simulink model "microturbine_model_v2"  (R2025b)
settings: Solver=ode4  StartTime=0.0  StopTime=inf  FixedStep=0.002  RelTol=1e-3
values from neighbouring files (symbols this model uses):
  c_p_air = 1005    [data_v2.m]
  c_p_eg = 1100    [data_v2.m]
  c_p_w = 4184    [data_v2.m]
  dp = dp_run    [data_v2.m]
  eps_HRB = 0.75    [data_v2.m]
  eta_c = 0.81    [data_v2.m]
  eta_comb = 0.99    [data_v2.m]
  eta_gen = 0.98    [data_v2.m]
  eta_mech = 0.97    [data_v2.m]
  eta_t = 0.88    [data_v2.m]
  hot_water_setpoint = 60    [data_v2.m]
  J = 3e-3    (= 0.003)    [data_v2.m]
  k_air = 1.4    [data_v2.m]
  lambda = 0.313    [data_v2.m]
  lambda_eg_filter = 15e3    (= 15000)    [data_v2.m]
  LHV = 47e6    (= 47000000)    [data_v2.m]
  M_buffer = 20    [data_v2.m]
  P0 = dp.power.P_el    [data_v2.m]
  P1 = P_amb - filter_P    (= 100325)    [data_v2.m]
  P_amb = 101325    [data_v2.m]
  P_el_max = 0.95 * max(sched.P_el_W)    [data_v2.m]
  P_el_min = 1.1 * polyval(fitPmin, T1 - 273.15) * 1e3    [data_v2.m]
  R_air = c_p_air * (k_air-1)/k_air    (= 287.142857143)    [data_v2.m]
  sched = sched_run    [data_v2.m]
  T1 = T1_run    (= 288.15)    [data_v2.m]
  T3_max = 960+273.15    (= 1233.15)    [data_v2.m]
  T3_min = 650+273.15    (= 923.15)    [data_v2.m]
  T_cold_water = 15    [data_v2.m]
  V = 0.025    [data_v2.m]
libraries: nesl_utility x4, simulink x3, slpidlib x2, fl_lib x1
settings Model: Creator=Alessandro  LastModifiedBy=Alessandro

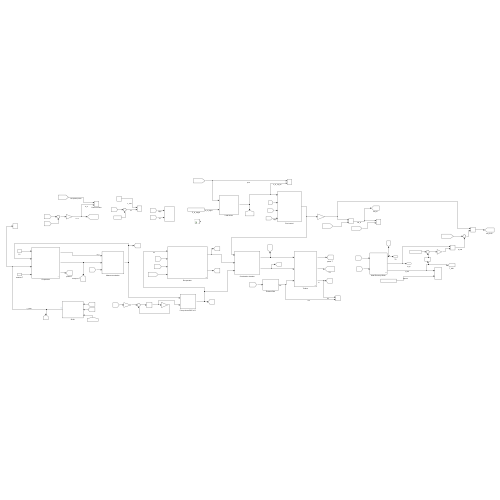
[thumbnail: Simulink's stored preview of the top-level diagram]
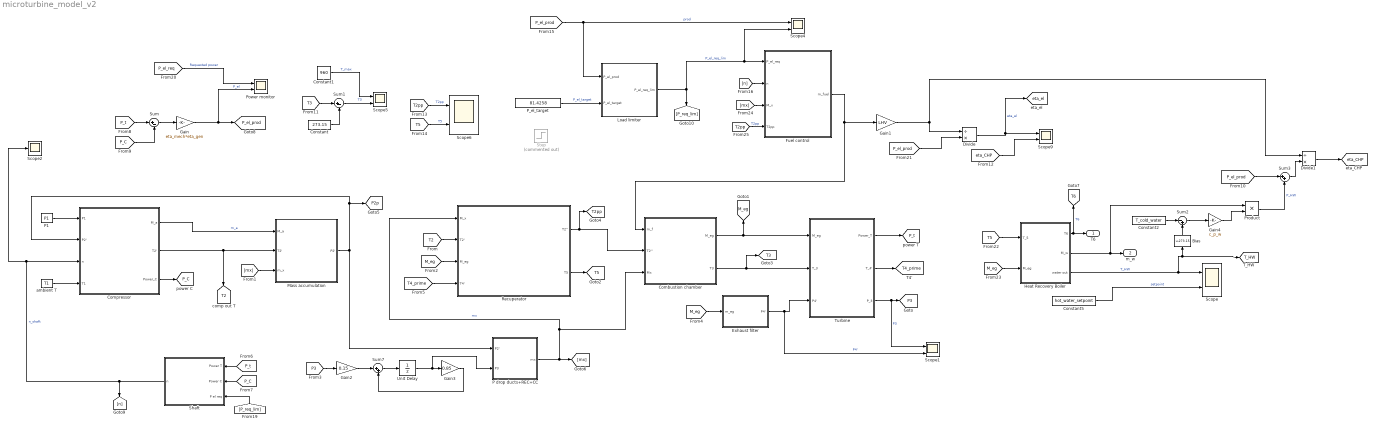
== system microturbine_model_v2 ==
  Bias : Bias  Bias=-273.15  SaturateOnIntegerOverflow=off
  Combustion chamber : Subsystem
      mask Display: image('360_F_235263034_miJw2igmixo7ymCqhHZ7c8wp9kaujzfM.jpg');
  Compressor : Subsystem
      mask Display: image('compressor_icon.png');
  Constant : Constant  Value=273.15
  Constant1 : Constant  Value=960
  Constant2 : Constant  Value=T_cold_water
  Constant5 : Constant  Value=hot_water_setpoint
  Divide : Product  Inputs=/*
  Divide1 : Product  Inputs=/*
  Exhaust filter : Subsystem
  Fuel control : Subsystem
  Gain : Gain  Gain=eta_mech*eta_gen
  Gain1 : Gain  Gain=LHV
  Gain2 : Gain  Gain=0.15
  Gain3 : Gain  Gain=0.85
  Gain4 : Gain  Gain=c_p_w
  Heat Recovery Boiler : Subsystem
  Load limiter : Subsystem
  Mass accumulation : Subsystem
  P drop ducts+REC+CC : Subsystem
  P1 : Constant  Value=P1
  P_el_target : Constant  Value=81.4258
  Power monitor : Scope  NumInputPorts=2
      settings: ActiveDisplayYMinimum=-9170.58872046804  ActiveDisplayYMaximum=119683.00366407538  DataLoggingDecimation=50  DataLoggingVariableName=ScopeData7
  Product : Product
  Recuperator : Subsystem
      mask Display: image('Heat-Transfer-in-a-Double-Pipe-Heat-Exchanger.jpg');
  Scope{,1,4..6,9} (6 alike) : Scope  NumInputPorts=2
      Scope settings: ActiveDisplayYMinimum=3.191503786041018  ActiveDisplayYMaximum=105.72122088980728  DataLoggingDecimation=50
      Scope1 settings: TimeDisplayOffset=20  ActiveDisplayYMinimum=-67410.697407891537  ActiveDisplayYMaximum=604536.71720488416  DataLoggingDecimation=50
      Scope4 settings: ActiveDisplayYMinimum=72643.782114693779  ActiveDisplayYMaximum=83704.868974122015  DataLoggingDecimation=50  DataLoggingVariableName=ScopeData8
      Scope5 settings: ActiveDisplayYMinimum=954.15751527655459  ActiveDisplayYMaximum=959.34960531631691  DataLoggingDecimation=50  DataLoggingVariableName=ScopeData5
      Scope6 settings: ActiveDisplayYMinimum=549.25379795566278  ActiveDisplayYMaximum=874.2834530892867  DataLoggingDecimation=50  DataLoggingVariableName=ScopeData6
      Scope9 settings: ActiveDisplayYMinimum=0.15948540822321575  ActiveDisplayYMaximum=0.4992395185212698  DataLoggingDecimation=50  DataLoggingVariableName=ScopeData9
  Scope2 : Scope
      settings: ActiveDisplayYMinimum=40436.974761073478  ActiveDisplayYMaximum=81944.16250433313  DataLoggingDecimation=50  DataLoggingVariableName=ScopeData2
  Shaft : Subsystem
  Step : Step  Commented=on  Time=10  Before=P0  After=P_el_max  SampleTime=0
  Sum : Sum  Inputs=|+-
  Sum1 : Sum  Inputs=|+-
  Sum2 : Sum  Inputs=|-+
  Sum3 : Sum  Inputs=|++
  Sum7 : Sum  Inputs=|++
  Turbine : Subsystem
  Unit Delay : UnitDelay  InitialCondition=dp.stations(3).P  SampleTime=-1  HasFrameUpgradeWarning=on
  ambient T : Constant  Value=T1
  T6 : Outport
  m_w : Outport  Port=2
  tag scope: M_eg=global, P2p=global, P3=global, P_C=global, P_el_prod=global, P_t=global, T2=global, T2pp=global, T3=global, T4_prime=global, T5=global, T6=global, T_HW=global, eta_CHP=global, eta_el=global
  wires:
  Compressor/1(M_a) -> Mass accumulation/1(M_a)  "m_a"
  Mass accumulation/1(P2') -> Compressor/2(P2'), [P2p], P drop ducts+REC+CC/1(P2')
  Compressor/2(T2') -> Mass accumulation/2(T2'), [T2]
  P1/1 -> Compressor/1(P1)
  [T2] -> Recuperator/2(T2')
  Recuperator/1(T2'') -> [T2pp], Combustion chamber/2("T2'' ")
  Combustion chamber/1("M_eg ") -> [M_eg], Turbine/1(M_eg)
  [M_eg] -> Recuperator/3(M_eg)
  Recuperator/2(T5) -> [T5]
  Combustion chamber/2(T3) -> [T3], Turbine/2(T_3)
  Turbine/3(P_3) -> Scope1/1, [P3]  "P3"
  Exhaust filter/1(P4') -> Scope1/2, Turbine/3(P4')  "P4'"
  [M_eg] -> Exhaust filter/1(m_eg)
  Compressor/3(Power_C) -> [P_C]
  [P_t] -> Shaft/1(Power T)
  [P_C] -> Shaft/2(Power C)
  [P_t] -> Sum/1
  [P_C] -> Sum/2
  Sum/1 -> Gain/1
  Gain/1 -> [P_el_prod], Power monitor/2  "P_el"
  P drop ducts+REC+CC/1(mx) -> [mx], Combustion chamber/3(Mx), Recuperator/1(M_x)  "mx"
  [mx] -> Mass accumulation/3(m_x)
  Fuel control/1(m_fuel) -> Combustion chamber/1(m_f), Gain1/1
  [P3] -> Gain2/1
  [T4_prime] -> Recuperator/4(T4')
  Turbine/2(T_4') -> [T4_prime]
  Turbine/1(Power_T) -> [P_t]
  Gain2/1 -> Sum7/1
  Unit Delay/1 -> P drop ducts+REC+CC/2(P3), Gain3/1
  Gain3/1 -> Sum7/2
  Sum7/1 -> Unit Delay/1
  [P_req_lim] -> Shaft/3(P el req)
  [T2pp] -> Scope6/1  "T2pp"
  [T5] -> Scope6/2  "T5"
  [T3] -> Sum1/1
  Sum1/1 -> Scope5/2  "T3"
  Constant/1 -> Sum1/2
  Constant1/1 -> Scope5/1  "T_max"
  [P_el_prod] -> Divide/2
  Gain1/1 -> Divide/1, Divide1/1
  Divide/1 -> [eta_el], Scope9/1  "eta_el"
  ambient T/1 -> Compressor/4(T1)
  [T5] -> Heat Recovery Boiler/1(T_5)
  [M_eg] -> Heat Recovery Boiler/2(M_eg)
  Heat Recovery Boiler/1(T6) -> T6/1, [T6]  "T6"
  Heat Recovery Boiler/2(M_w) -> Product/1, m_w/1
  Heat Recovery Boiler/3(water out) -> Bias/1, [T_HW], Scope/1  "T_HW"
  Constant5/1 -> Scope/2  "setpoint"
  [P_el_req] -> Power monitor/1  "Requested power"
  [mx] -> Fuel control/3(M_x)
  [T2pp] -> Fuel control/4(T2pp)  "T2pp"
  [n] -> Fuel control/2(n)
  [P_el_prod] -> Load limiter/1(P_el_prod), Scope4/1  "prod"
  Shaft/1(n) -> Scope2/1, Compressor/3(n), [n]  "n_shaft"
  Load limiter/1(P_el_req_lim) -> [P_req_lim], Scope4/2, Fuel control/1(P_el_req)  "P_el_req_lim"
  P_el_target/1 -> Load limiter/2(P_el_target)  "P_el_target"
  Constant2/1 -> Sum2/1
  Sum2/1 -> Gain4/1
  Gain4/1 -> Product/2
  Product/1 -> Sum3/2  "P_HW"
  [P_el_prod] -> Sum3/1
  Sum3/1 -> Divide1/2
  Divide1/1 -> [eta_CHP]
  [eta_CHP] -> Scope9/2
  Bias/1 -> Sum2/2

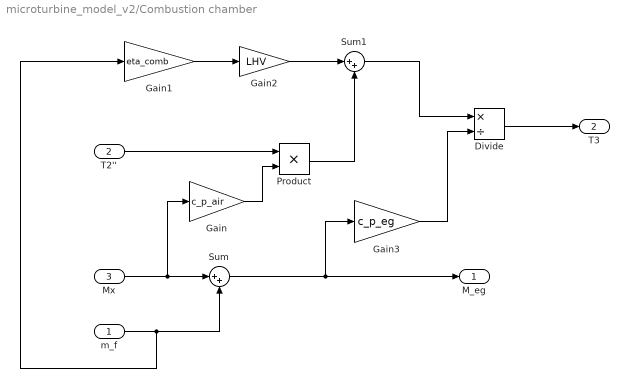
== system microturbine_model_v2/Combustion chamber ==
  m_f : Inport
  "T2'' " : Inport  Port=2
  Mx : Inport  Port=3
  Divide : Product  Inputs=*/
  Gain : Gain  Gain=c_p_air
  Gain1 : Gain  Gain=eta_comb
  Gain2 : Gain  Gain=LHV
  Gain3 : Gain  Gain=c_p_eg
  Product : Product
  Sum : Sum  Inputs=|++
  Sum1 : Sum  Inputs=|++
  "M_eg " : Outport
  T3 : Outport  Port=2
  wires:
  Sum/1 -> "M_eg "/1, Gain3/1
  Mx/1 -> Gain/1, Sum/1
  m_f/1 -> Sum/2, Gain1/1
  Sum1/1 -> Divide/1
  Divide/1 -> T3/1
  Gain/1 -> Product/2
  Gain1/1 -> Gain2/1
  Gain2/1 -> Sum1/1
  "T2'' "/1 -> Product/1
  Product/1 -> Sum1/2
  Gain3/1 -> Divide/2

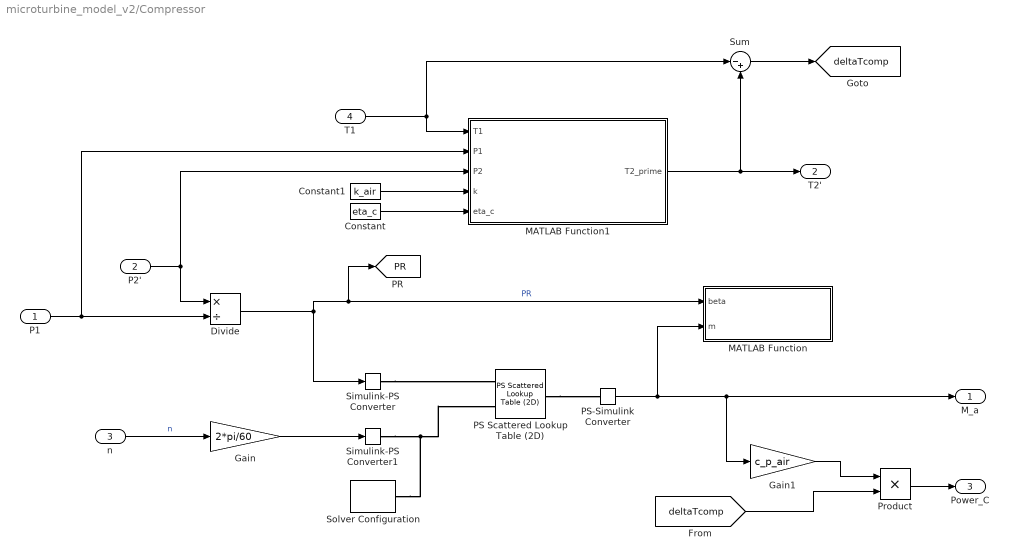
== system microturbine_model_v2/Compressor ==
  P1 : Inport
  P2' : Inport  Port=2
  n : Inport  Port=3
  T1 : Inport  Port=4
  Constant : Constant  Value=eta_c
  Constant1 : Constant  Value=k_air
  Divide : Product  Inputs=*/
  Gain : Gain  Gain=2*pi/60
  Gain1 : Gain  Gain=c_p_air
  MATLAB Function : MATLAB Function  TreatAsAtomicUnit=on
  MATLAB Function1 : MATLAB Function  TreatAsAtomicUnit=on
  PS Scattered Lookup Table (2D) : fl_lib/Physical Signals/Lookup Tables/PS Scattered Lookup Table (2D)  x1=beta  x2=n rad/s  f=flow kg/s  extrap_method=simscape.enum.extrapolation_slu.linear
      settings: InternalSimscapePortConfiguration="{\"Bottom\":[],\"Left\":[{\"id\":\"I1\",\"label\":\"x1\",\"type\":\"input\"},{\"id\":\"I2\",\"label\":\"x2\",\"type\":\"input\"}],\"Right\":[{\"id\":\"O\",\"label\":\"f\",\"type\":\"output\"}],\"Top\":[]}"
  PS-Simulink Converter : nesl_utility/PS-Simulink Converter  PhysicalDomain=network_engine_domain  SubClassName=ps_output  LeftPortType=input  RightPortType=output  PseudoPeriodic=off  Frequencies=[]  VectorFormat=inherit  Unit=inherit  AffineConversion=off
  Product : Product
  Simulink-PS Converter : nesl_utility/Simulink-PS Converter  PhysicalDomain=network_engine_domain  SubClassName=ps_input  LeftPortType=input  RightPortType=output  PseudoPeriodic=off  Frequencies=[]  NoiseDistribution=none  NoiseParameters=[]  Unit=1  AffineConversion=off  FilteringAndDerivatives=provide  SimscapeFilterOrder=1  InputFilterTimeConstant=0.001  UdotUserProvided=0
  Simulink-PS Converter1 : nesl_utility/Simulink-PS Converter  PhysicalDomain=network_engine_domain  SubClassName=ps_input  LeftPortType=input  RightPortType=output  PseudoPeriodic=off  Frequencies=[]  NoiseDistribution=none  NoiseParameters=[]  Unit=rad/s  AffineConversion=off  FilteringAndDerivatives=provide  SimscapeFilterOrder=1  InputFilterTimeConstant=0.001  UdotUserProvided=0
  Solver Configuration : nesl_utility/Solver Configuration  PhysicalDomain=network_engine_domain  SubClassName=solver  LeftPortType=input  RightPortType=generic  Tones=[]  Harmonics=[]  SimulateNoise=off  Profile=off  UseLocalSampling=off  EnableSwitchedLinearOptims=on  FrequencyDomain=off  UseCCode=off  RelTol=0.001  AbsTol=0.001  MinStep=1e-09  ToWorkspace=off  RevertToSquareIcSolve=off  NumHomotopyIterations=100  PhasorMode=off  PhasorModeNumHarmonics=1  ConsistencySolver=NEWTON_XTOL_AFTER_FTOL  IndexReductionMethod=DerivativeReplacement  DoDC=off  ResidualTolerance=1e-09  ConsistencyTolSource=GLOBAL  ConsistencyAbsTol=0.001  ConsistencyRelTol=0.001  ConsistencyTolFactor=0.001  UseLocalSolver=off  LocalSolverChoice=NE_BACKWARD_EULER_ADVANCER  ResolveIndetEquations=on  FunctionEvalNumThread=1  LocalSolverSampleTime=0.0001  DoFixedCost=off  MaxNonlinIter=3  MaxModeIter=2  ComputeImpulses=off  ImpulseIterations=2  LinearAlgebra=auto  LinearAlgebraNumThread=0  EquationFormulation=NE_TIME_EF  DelaysMemoryBudget=1024  AutomaticFiltering=on  FilteringTimeConstant=0.001  PartitionStorageMethod=AS_NEEDED  PartitionMemoryBudget=1024  PartitionMethod=ROBUST  MultibodyUseLocalSolver=off  MultibodyLocalSolverChoice=ODE1  MultibodyLocalSolverSampleTime=0.001
  Sum : Sum  Inputs=|-+
  M_a : Outport
  T2' : Outport  Port=2
  Power_C : Outport  Port=3
  tag scope: PR=global, deltaTcomp=global
  wires:
  PS-Simulink Converter/1 -> MATLAB Function/2(m), Gain1/1, M_a/1
  Gain/1 -> Simulink-PS Converter1/1
  n/1 -> Gain/1  "n"
  P2'/1 -> MATLAB Function1/3(P2), Divide/1
  P1/1 -> MATLAB Function1/2(P1), Divide/2
  Divide/1 -> Simulink-PS Converter/1, [PR], MATLAB Function/1(beta)  "PR"
  Constant1/1 -> MATLAB Function1/4(k)
  T1/1 -> MATLAB Function1/1(T1), Sum/1
  Constant/1 -> MATLAB Function1/5(eta_c)
  MATLAB Function1/1(T2_prime) -> Sum/2, T2'/1
  Sum/1 -> [deltaTcomp]
  Gain1/1 -> Product/1
  [deltaTcomp] -> Product/2
  Product/1 -> Power_C/1
  connections:
  Simulink-PS Converter/RConn1 -- PS Scattered Lookup Table (2D)/LConn1
  Simulink-PS Converter1/RConn1 -- PS Scattered Lookup Table (2D)/LConn2 -- Solver Configuration/RConn1
  PS Scattered Lookup Table (2D)/RConn1 -- PS-Simulink Converter/LConn1

== system microturbine_model_v2/Exhaust filter ==
  m_eg : Inport
  Constant1 : Constant  Value=P_amb
  Gain : Gain  Gain=lambda_eg_filter
  Square : Math  Operator=square
  Sum : Sum  Inputs=|++
  P4' : Outport
  wires:
  Gain/1 -> Sum/1
  Constant1/1 -> Sum/2
  Square/1 -> Gain/1
  Sum/1 -> P4'/1
  m_eg/1 -> Square/1

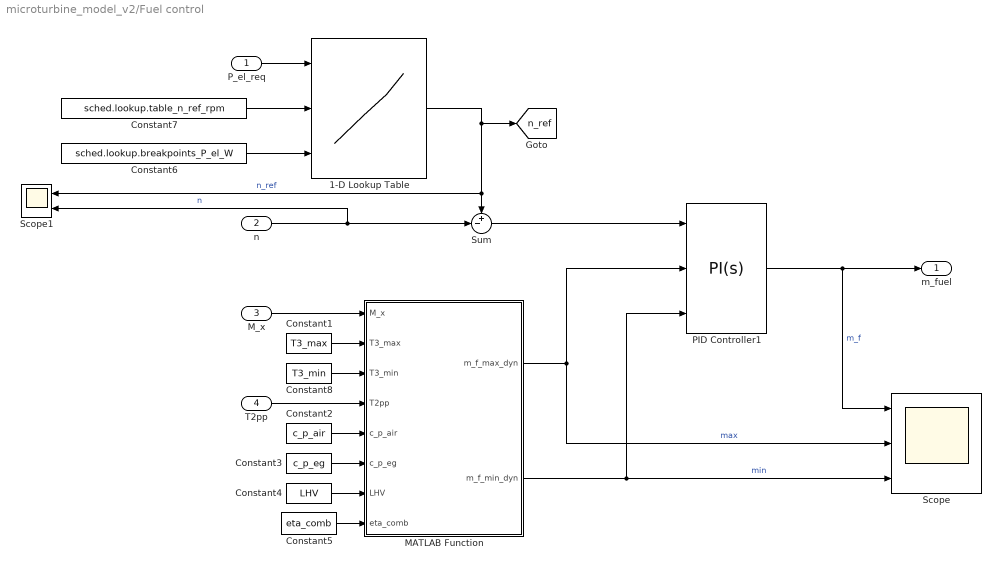
== system microturbine_model_v2/Fuel control ==
  P_el_req : Inport
  n : Inport  Port=2
  M_x : Inport  Port=3
  T2pp : Inport  Port=4
  1-D Lookup Table : Lookup_n-D  NumberOfTableDimensions=1  BreakpointsForDimension1Source=Input port  BreakpointsForDimension1=[-5:5]  BeginIndexSearchUsingPreviousIndexResult=on  TableSource=Input port  Table=tanh([-5:5])  ExtrapMethod=Clip  DiagnosticForOutOfRangeInput=Warning  InternalRulePriority=Speed  RndMeth=Simplest
      settings: InputPortMap=u0,p221,p5
  Constant1 : Constant  Value=T3_max
  Constant2 : Constant  Value=c_p_air
  Constant3 : Constant  Value=c_p_eg
  Constant4 : Constant  Value=LHV
  Constant5 : Constant  Value=eta_comb
  Constant6 : Constant  Value=sched.lookup.breakpoints_P_el_W
  Constant7 : Constant  Value=sched.lookup.table_n_ref_rpm
  Constant8 : Constant  Value=T3_min
  MATLAB Function : MATLAB Function  TreatAsAtomicUnit=on
  PID Controller1 : slpidlib/PID Controller  Controller=PI  Form=Parallel  TimeDomain=Continuous-time  UseExternalTs=off  SampleTime=-1  IntegratorMethod=Forward Euler  FilterMethod=Forward Euler  ControllerParametersSource=internal  P=4e-7  I=1.5e-7  UseKiTs=off  D=0  UseExternalDerivativeSource=off  N=100  UseFilter=on  TunerSelectOption=Transfer Function Based (PID Tuner App)  InitialConditionSource=internal  InitialConditionForIntegrator=dp.m_fuel  InitialConditionForFilter=0  DifferentiatorICPrevScaledInput=0  ExternalReset=none  TrackingMode=off  Kt=1  LimitOutput=on  SatLimitsSource=external  UpperSaturationLimit=0.01  LowerSaturationLimit=0  LinearizeAsGain=on  AntiWindupMode=clamping  Kb=1  LimitIntegrator=off  UpperIntegratorSaturationLimit=inf  LowerIntegratorSaturationLimit=-inf  POutMin=[]  POutMax=[]  IOutMin=[]  IOutMax=[]  DOutMin=[]  DOutMax=[]  NOutMin=[]  NOutMax=[]  SumOutMin=[]  SumOutMax=[]  SaturationOutMin=[]  SaturationOutMax=[]  PParamMin=[]  PParamMax=[]  IParamMin=[]  IParamMax=[]  DParamMin=[]  DParamMax=[]  NParamMin=[]  NParamMax=[]  KbParamMin=[]  KbParamMax=[]  KtParamMin=[]  KtParamMax=[]  KbOutMin=[]  KbOutMax=[]  KtOutMin=[]  KtOutMax=[]  IntegratorOutMin=[]  IntegratorOutMax=[]  FilterOutMin=[]  FilterOutMax=[]  SumI1OutMin=[]  SumI1OutMax=[]  SumI2OutMin=[]  SumI2OutMax=[]  SumI3OutMin=[]  SumI3OutMax=[]  SumI4OutMin=[]  SumI4OutMax=[]  SumDOutMin=[]  SumDOutMax=[]  DifferentiatorOutMin=[]  DifferentiatorOutMax=[]  FilterDiffOutCoefMin=[]  FilterDiffOutCoefMax=[]  ReciprocalOutMin=[]  ReciprocalOutMax=[]  SumDenOutMin=[]  SumDenOutMax=[]  SumNumOutMin=[]  SumNumOutMax=[]  DivideOutMin=[]  DivideOutMax=[]  UdiffTsProdOutMin=[]  UdiffTsProdOutMax=[]  NTsProdOutMin=[]  NTsProdOutMax=[]  UintegralTsProdOutMin=[]  UintegralTsProdOutMax=[]  UngainTsProdOutMin=[]  UngainTsProdOutMax=[]  ClampingZeroOutDataTypeStr=Inherit: Inherit via back propagation  ClampingZeroOutMin=[]  ClampingZeroOutMax=[]  FilterDenConstantOutDataTypeStr=Inherit: Inherit via back propagation  FilterDenConstantOutMin=[]  FilterDenConstantOutMax=[]  PCopyOutDataTypeStr=Inherit: Inherit via back propagation  PCopyOutMin=[]  PCopyOutMax=[]  NCopyOutDataTypeStr=Inherit: Inherit via back propagation  NCopyOutMin=[]  NCopyOutMax=[]  IntegratorContinuousStateAttributes=''  IntegratorStateMustResolveToSignalObject=off  IntegratorRTWStateStorageClass=Auto  FilterContinuousStateAttributes=''  FilterStateMustResolveToSignalObject=off  FilterRTWStateStorageClass=Auto  ParallelPVariant=InternalParameters  IdealPVariant=Disabled  IVariant=InternalParameters  DVariant=Disabled  IntegratorVariant=Continuous  SatVariant=External  AWVariant=ContClampingParallel  PCopyVariant=Disabled  TRVariant=Disabled  FdbkBlocksVariant=Forward  IdealPFdbkVariant=Disabled  SatFdbkVariant=Disabled  DerivativeFilterVariant=Disabled  NVariant=Disabled  NCopyVariant=Disabled_SignalSpec  FilterICVariant=Disabled  IntegratorICVariant=InternalICs  ExternalResetVariant=Disabled  TRSumVariant=Passthrough  SumFdbkVariant=Disabled  SumVariant=Sum_PI  TsampFilterVariant=InternalTs  TsampNgainVariant=Passthrough  TsampIntegralVariant=Disabled_SignalSpec  ExternalSaturationOutDataTypeStr=Inherit: Same as second input  DerivativeSourceVariant=Disabled  PreIntVariant=InternalPreInt
  Scope : Scope  NumInputPorts=3
      settings: TimeDisplayOffset=20  ActiveDisplayYMinimum=0.0026657090990522842  ActiveDisplayYMaximum=0.0086392131535926436  DataLoggingDecimation=50  DataLoggingVariableName=ScopeData10
  Scope1 : Scope  NumInputPorts=2
      settings: ActiveDisplayYMinimum=57626.38447332372  ActiveDisplayYMaximum=65305.577790295967  DataLoggingDecimation=50  DataLoggingVariableName=ScopeData12
  Sum : Sum  Inputs=+-|
  m_fuel : Outport
  tag scope: n_ref=global
  wires:
  M_x/1 -> MATLAB Function/1(M_x)
  Constant1/1 -> MATLAB Function/2(T3_max)
  T2pp/1 -> MATLAB Function/4(T2pp)
  Constant2/1 -> MATLAB Function/5(c_p_air)
  Constant3/1 -> MATLAB Function/6(c_p_eg)
  Constant4/1 -> MATLAB Function/7(LHV)
  Constant5/1 -> MATLAB Function/8(eta_comb)
  MATLAB Function/1(m_f_max_dyn) -> PID Controller1/2, Scope/2  "max"
  PID Controller1/1 -> Scope/1, m_fuel/1  "m_f"
  n/1 -> Scope1/2, Sum/2  "n"
  P_el_req/1 -> 1-D Lookup Table/1
  Constant6/1 -> 1-D Lookup Table/3
  Constant7/1 -> 1-D Lookup Table/2
  1-D Lookup Table/1 -> [n_ref], Scope1/1, Sum/1  "n_ref"
  Sum/1 -> PID Controller1/1
  Constant8/1 -> MATLAB Function/3(T3_min)
  MATLAB Function/2(m_f_min_dyn) -> PID Controller1/3, Scope/3  "min"

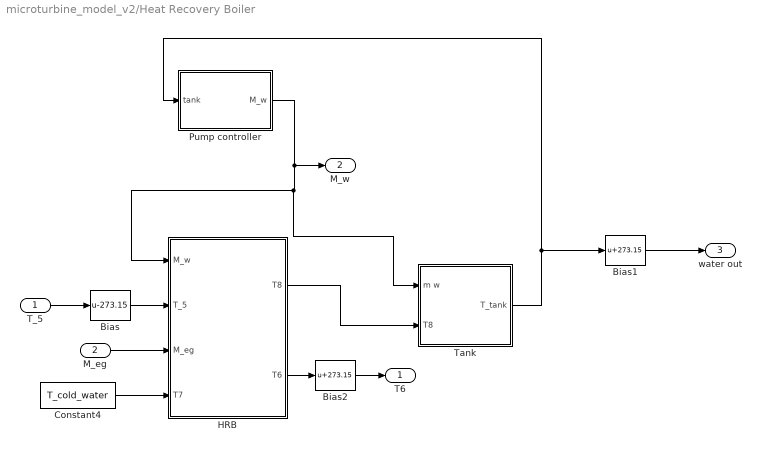
== system microturbine_model_v2/Heat Recovery Boiler ==
  T_5 : Inport
  M_eg : Inport  Port=2
  Bias : Bias  Bias=-273.15  SaturateOnIntegerOverflow=off
  Bias1 : Bias  Bias=273.15  SaturateOnIntegerOverflow=off
  Bias2 : Bias  Bias=273.15  SaturateOnIntegerOverflow=off
  Constant4 : Constant  Value=T_cold_water
  HRB : Subsystem
  Pump controller : Subsystem
  Tank : Subsystem
  T6 : Outport
  M_w : Outport  Port=2
  water out : Outport  Port=3
  wires:
  Bias/1 -> HRB/2(T_5)
  T_5/1 -> Bias/1
  HRB/2(T6) -> Bias2/1
  M_eg/1 -> HRB/3(M_eg)
  Constant4/1 -> HRB/4(T7)
  Pump controller/1(M_w) -> M_w/1, Tank/1(m w), HRB/1(M_w)
  HRB/1(T8) -> Tank/2(T8)
  Tank/1(T_tank) -> Bias1/1, Pump controller/1(tank)
  Bias2/1 -> T6/1
  Bias1/1 -> water out/1

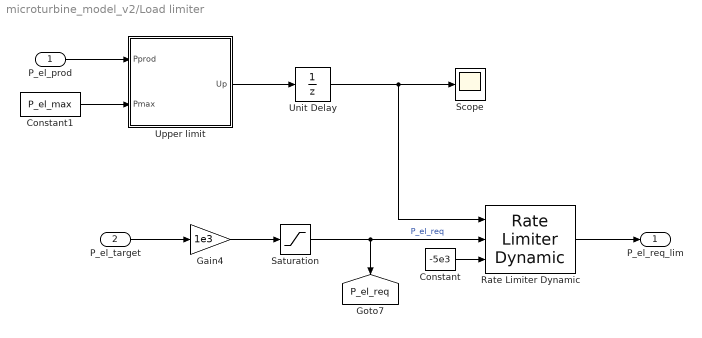
== system microturbine_model_v2/Load limiter ==
  P_el_prod : Inport
  P_el_target : Inport  Port=2
  Constant : Constant  Value=-5e3
  Constant1 : Constant  Value=P_el_max
  Gain4 : Gain  Gain=1e3
  Rate Limiter Dynamic : simulink/Discontinuities/Rate Limiter Dynamic
  Saturation : Saturate  UpperLimit=P_el_max  LowerLimit=P_el_min
  Scope : Scope
      settings: ActiveDisplayYMinimum=99.299018908265339  ActiveDisplayYMaximum=132.72806509392043  DataLoggingDecimation=50  DataLoggingVariableName=ScopeData3
  Unit Delay : UnitDelay  InitialCondition=700  SampleTime=-1  HasFrameUpgradeWarning=on
  Upper limit : MATLAB Function  TreatAsAtomicUnit=on
  P_el_req_lim : Outport
  tag scope: P_el_req=global
  wires:
  Saturation/1 -> [P_el_req], Rate Limiter Dynamic/2  "P_el_req"
  P_el_target/1 -> Gain4/1
  Gain4/1 -> Saturation/1
  Rate Limiter Dynamic/1 -> P_el_req_lim/1
  Constant/1 -> Rate Limiter Dynamic/3
  Constant1/1 -> Upper limit/2(Pmax)
  P_el_prod/1 -> Upper limit/1(Pprod)
  Upper limit/1(Up) -> Unit Delay/1
  Unit Delay/1 -> Scope/1, Rate Limiter Dynamic/1

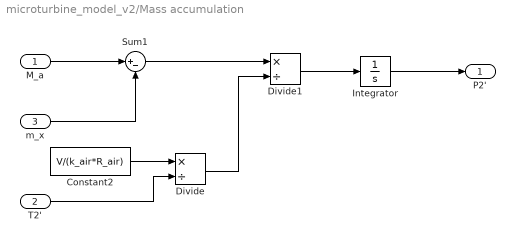
== system microturbine_model_v2/Mass accumulation ==
  M_a : Inport
  T2' : Inport  Port=2
  m_x : Inport  Port=3
  Constant2 : Constant  Value=V/(k_air*R_air)
  Divide : Product  Inputs=*/
  Divide1 : Product  Inputs=*/
  Integrator : Integrator  InitialCondition=dp.stations(2).P
  Sum1 : Sum  Inputs=|+-
  P2' : Outport
  wires:
  M_a/1 -> Sum1/1
  Sum1/1 -> Divide1/1
  Divide/1 -> Divide1/2
  Integrator/1 -> P2'/1
  Constant2/1 -> Divide/1
  T2'/1 -> Divide/2
  Divide1/1 -> Integrator/1
  m_x/1 -> Sum1/2

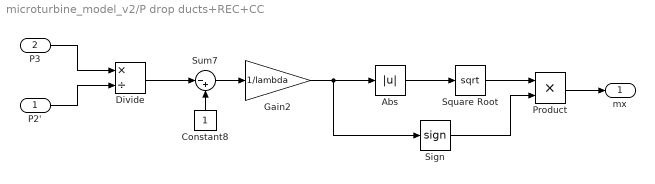
== system microturbine_model_v2/P drop ducts+REC+CC ==
  P2' : Inport
  P3 : Inport  Port=2
  Abs : Abs  SaturateOnIntegerOverflow=off
  Constant8 : Constant
  Divide : Product  Inputs=*/
  Gain2 : Gain  Gain=1/lambda
  Product : Product
  Sign : Signum
  Square Root : Sqrt
  Sum7 : Sum  Inputs=|-+
  mx : Outport
  wires:
  Constant8/1 -> Sum7/2
  P2'/1 -> Divide/2
  P3/1 -> Divide/1
  Sum7/1 -> Gain2/1
  Gain2/1 -> Sign/1, Abs/1
  Divide/1 -> Sum7/1
  Abs/1 -> Square Root/1
  Square Root/1 -> Product/1
  Sign/1 -> Product/2
  Product/1 -> mx/1

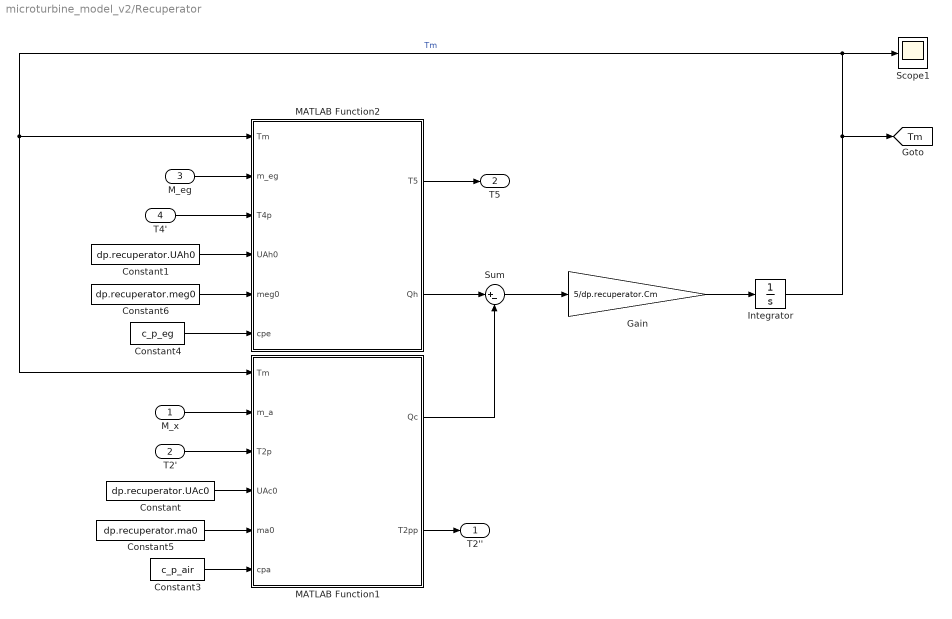
== system microturbine_model_v2/Recuperator ==
  M_x : Inport
  T2' : Inport  Port=2
  M_eg : Inport  Port=3
  T4' : Inport  Port=4
  Constant : Constant  Value=dp.recuperator.UAc0
  Constant1 : Constant  Value=dp.recuperator.UAh0
  Constant3 : Constant  Value=c_p_air
  Constant4 : Constant  Value=c_p_eg
  Constant5 : Constant  Value=dp.recuperator.ma0
  Constant6 : Constant  Value=dp.recuperator.meg0
  Gain : Gain  Gain=5/dp.recuperator.Cm
  Integrator : Integrator  InitialCondition=dp.recuperator.Tm0
  MATLAB Function1 : MATLAB Function  TreatAsAtomicUnit=on
  MATLAB Function2 : MATLAB Function  TreatAsAtomicUnit=on
  Scope1 : Scope
      settings: ActiveDisplayYMinimum=388.65870173537724  ActiveDisplayYMaximum=864.02305810409723  DataLoggingDecimation=50  DataLoggingVariableName=ScopeData11
  Sum : Sum  Inputs=|+-
  T2'' : Outport
  T5 : Outport  Port=2
  tag scope: Tm=global
  wires:
  Integrator/1 -> Scope1/1, MATLAB Function2/1(Tm), MATLAB Function1/1(Tm), [Tm]  "Tm"
  MATLAB Function2/1(T5) -> T5/1
  MATLAB Function1/2(T2pp) -> T2''/1
  Constant3/1 -> MATLAB Function1/6(cpa)
  Constant5/1 -> MATLAB Function1/5(ma0)
  Constant/1 -> MATLAB Function1/4(UAc0)
  Constant4/1 -> MATLAB Function2/6(cpe)
  Constant1/1 -> MATLAB Function2/4(UAh0)
  T4'/1 -> MATLAB Function2/3(T4p)
  M_eg/1 -> MATLAB Function2/2(m_eg)
  M_x/1 -> MATLAB Function1/2(m_a)
  T2'/1 -> MATLAB Function1/3(T2p)
  Constant6/1 -> MATLAB Function2/5(meg0)
  MATLAB Function2/2(Qh) -> Sum/1
  MATLAB Function1/1(Qc) -> Sum/2
  Sum/1 -> Gain/1
  Gain/1 -> Integrator/1

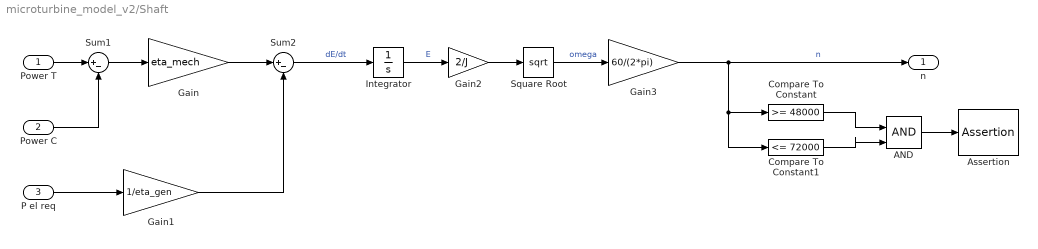
== system microturbine_model_v2/Shaft ==
  Power T : Inport
  Power C : Inport  Port=2
  P el req : Inport  Port=3
  AND : Logic  IconShape=distinctive  AllPortsSameDT=off  OutDataTypeStr=boolean
  Assertion : Assertion  AssertionFailFcn=shaft speed outside of compressor map validity range
  Compare To Constant : simulink/Logic and Bit Operations/Compare To Constant  relop=>=  const=48000  OutDataTypeStr=boolean
  Compare To Constant1 : simulink/Logic and Bit Operations/Compare To Constant  relop=<=  const=72000  OutDataTypeStr=boolean
  Gain : Gain  Gain=eta_mech
  Gain1 : Gain  Gain=1/eta_gen
  Gain2 : Gain  Gain=2/J
  Gain3 : Gain  Gain=60/(2*pi)
  Integrator : Integrator  InitialCondition=dp.shaft.kinEn
  Square Root : Sqrt
  Sum1 : Sum  Inputs=|+-
  Sum2 : Sum  Inputs=|+-
  n : Outport
  wires:
  Sum1/1 -> Gain/1
  Power C/1 -> Sum1/2
  Integrator/1 -> Gain2/1  "E"
  P el req/1 -> Gain1/1
  Power T/1 -> Sum1/1
  Square Root/1 -> Gain3/1  "omega"
  Sum2/1 -> Integrator/1  "dE/dt"
  Gain3/1 -> Compare To Constant1/1, Compare To Constant/1, n/1  "n"
  Gain2/1 -> Square Root/1
  Gain1/1 -> Sum2/2
  Gain/1 -> Sum2/1
  AND/1 -> Assertion/1
  Compare To Constant/1 -> AND/1
  Compare To Constant1/1 -> AND/2

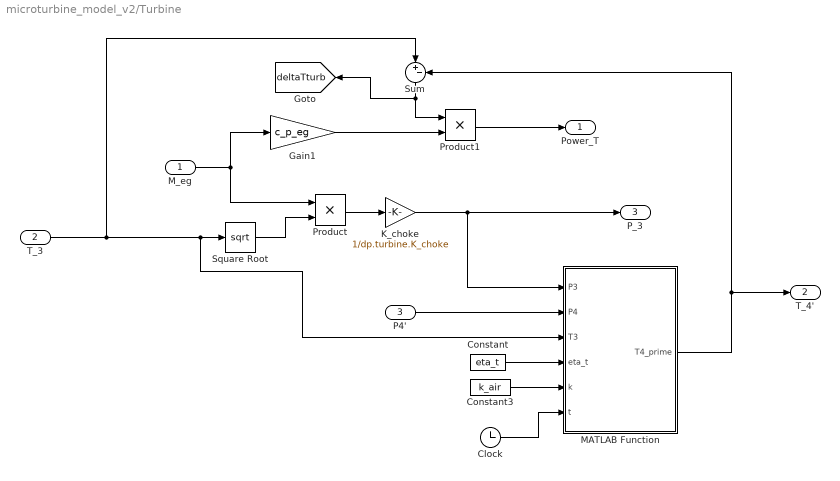
== system microturbine_model_v2/Turbine ==
  M_eg : Inport
  T_3 : Inport  Port=2
  P4' : Inport  Port=3
  Clock : Clock
  Constant : Constant  Value=eta_t
  Constant3 : Constant  Value=k_air
  Gain1 : Gain  Gain=c_p_eg
  K_choke : Gain  Gain=1/dp.turbine.K_choke
  MATLAB Function : MATLAB Function  TreatAsAtomicUnit=on
  Product : Product
  Product1 : Product
  Square Root : Sqrt
  Sum : Sum  Inputs=|+-
  Power_T : Outport
  T_4' : Outport  Port=2
  P_3 : Outport  Port=3
  tag scope: deltaTturb=global
  wires:
  K_choke/1 -> MATLAB Function/1(P3), P_3/1
  T_3/1 -> Sum/1, MATLAB Function/3(T3), Square Root/1
  M_eg/1 -> Product/1, Gain1/1
  Constant/1 -> MATLAB Function/4(eta_t)
  Square Root/1 -> Product/2
  Product/1 -> K_choke/1
  P4'/1 -> MATLAB Function/2(P4)
  MATLAB Function/1(T4_prime) -> Sum/2, T_4'/1
  Constant3/1 -> MATLAB Function/5(k)
  Gain1/1 -> Product1/2
  Sum/1 -> [deltaTturb], Product1/1
  Product1/1 -> Power_T/1
  Clock/1 -> MATLAB Function/6(t)

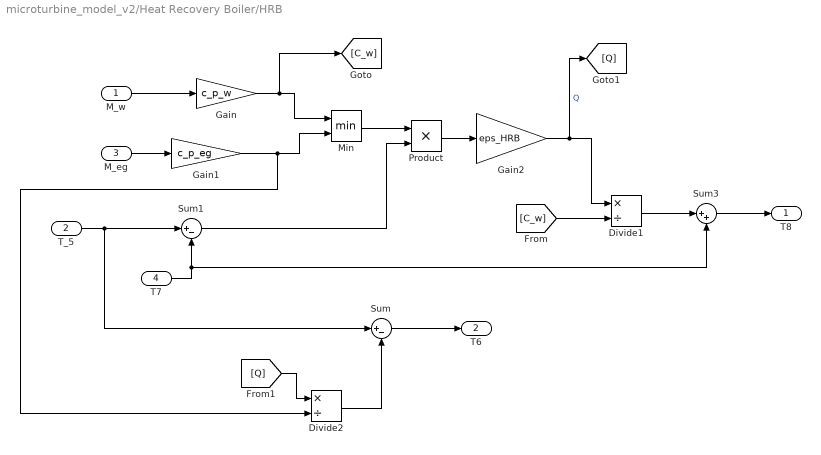
== system microturbine_model_v2/Heat Recovery Boiler/HRB ==
  M_w : Inport
  T_5 : Inport  Port=2
  M_eg : Inport  Port=3
  T7 : Inport  Port=4
  Divide1 : Product  Inputs=*/
  Divide2 : Product  Inputs=*/
  Gain : Gain  Gain=c_p_w
  Gain1 : Gain  Gain=c_p_eg
  Gain2 : Gain  Gain=eps_HRB
  Min : MinMax  Inputs=2
  Product : Product
  Sum : Sum  Inputs=|+-
  Sum1 : Sum  Inputs=|+-
  Sum3 : Sum  Inputs=|++
  T8 : Outport
  T6 : Outport  Port=2
  wires:
  Sum1/1 -> Product/2
  T_5/1 -> Sum/1, Sum1/1
  Sum3/1 -> T8/1
  T7/1 -> Sum3/2, Sum1/2
  Gain2/1 -> [Q], Divide1/1  "Q"
  Divide1/1 -> Sum3/1
  M_eg/1 -> Gain1/1
  Gain/1 -> [C_w], Min/1
  Gain1/1 -> Divide2/2, Min/2
  Product/1 -> Gain2/1
  M_w/1 -> Gain/1
  Min/1 -> Product/1
  [C_w] -> Divide1/2
  [Q] -> Divide2/1
  Divide2/1 -> Sum/2
  Sum/1 -> T6/1

== system microturbine_model_v2/Heat Recovery Boiler/Pump controller ==
  tank : Inport
  Constant : Constant  Value=hot_water_setpoint
  PID Controller : slpidlib/PID Controller  Controller=PI  Form=Parallel  TimeDomain=Continuous-time  UseExternalTs=off  SampleTime=-1  IntegratorMethod=Forward Euler  FilterMethod=Forward Euler  ControllerParametersSource=internal  P=0.06  I=5e-3  UseKiTs=off  D=0  UseExternalDerivativeSource=off  N=100  UseFilter=on  TunerSelectOption=Transfer Function Based (PID Tuner App)  InitialConditionSource=internal  InitialConditionForIntegrator=m_w_des  InitialConditionForFilter=0  DifferentiatorICPrevScaledInput=0  ExternalReset=none  TrackingMode=off  Kt=1  LimitOutput=on  SatLimitsSource=internal  UpperSaturationLimit=1.5  LowerSaturationLimit=0.01  LinearizeAsGain=on  AntiWindupMode=clamping  Kb=1  LimitIntegrator=off  UpperIntegratorSaturationLimit=inf  LowerIntegratorSaturationLimit=-inf  POutMin=[]  POutMax=[]  IOutMin=[]  IOutMax=[]  DOutMin=[]  DOutMax=[]  NOutMin=[]  NOutMax=[]  SumOutMin=[]  SumOutMax=[]  SaturationOutMin=[]  SaturationOutMax=[]  PParamMin=[]  PParamMax=[]  IParamMin=[]  IParamMax=[]  DParamMin=[]  DParamMax=[]  NParamMin=[]  NParamMax=[]  KbParamMin=[]  KbParamMax=[]  KtParamMin=[]  KtParamMax=[]  KbOutMin=[]  KbOutMax=[]  KtOutMin=[]  KtOutMax=[]  IntegratorOutMin=[]  IntegratorOutMax=[]  FilterOutMin=[]  FilterOutMax=[]  SumI1OutMin=[]  SumI1OutMax=[]  SumI2OutMin=[]  SumI2OutMax=[]  SumI3OutMin=[]  SumI3OutMax=[]  SumI4OutMin=[]  SumI4OutMax=[]  SumDOutMin=[]  SumDOutMax=[]  DifferentiatorOutMin=[]  DifferentiatorOutMax=[]  FilterDiffOutCoefMin=[]  FilterDiffOutCoefMax=[]  ReciprocalOutMin=[]  ReciprocalOutMax=[]  SumDenOutMin=[]  SumDenOutMax=[]  SumNumOutMin=[]  SumNumOutMax=[]  DivideOutMin=[]  DivideOutMax=[]  UdiffTsProdOutMin=[]  UdiffTsProdOutMax=[]  NTsProdOutMin=[]  NTsProdOutMax=[]  UintegralTsProdOutMin=[]  UintegralTsProdOutMax=[]  UngainTsProdOutMin=[]  UngainTsProdOutMax=[]  ClampingZeroOutDataTypeStr=Inherit: Inherit via back propagation  ClampingZeroOutMin=[]  ClampingZeroOutMax=[]  FilterDenConstantOutDataTypeStr=Inherit: Inherit via back propagation  FilterDenConstantOutMin=[]  FilterDenConstantOutMax=[]  PCopyOutDataTypeStr=Inherit: Inherit via back propagation  PCopyOutMin=[]  PCopyOutMax=[]  NCopyOutDataTypeStr=Inherit: Inherit via back propagation  NCopyOutMin=[]  NCopyOutMax=[]  IntegratorContinuousStateAttributes=''  IntegratorStateMustResolveToSignalObject=off  IntegratorRTWStateStorageClass=Auto  FilterContinuousStateAttributes=''  FilterStateMustResolveToSignalObject=off  FilterRTWStateStorageClass=Auto  ParallelPVariant=InternalParameters  IdealPVariant=Disabled  IVariant=InternalParameters  DVariant=Disabled  IntegratorVariant=Continuous  SatVariant=Enabled  AWVariant=ContClampingParallel  PCopyVariant=Disabled  TRVariant=Disabled  FdbkBlocksVariant=Forward  IdealPFdbkVariant=Disabled  SatFdbkVariant=Disabled  DerivativeFilterVariant=Disabled  NVariant=Disabled  NCopyVariant=Disabled_SignalSpec  FilterICVariant=Disabled  IntegratorICVariant=InternalICs  ExternalResetVariant=Disabled  TRSumVariant=Passthrough  SumFdbkVariant=Disabled  SumVariant=Sum_PI  TsampFilterVariant=InternalTs  TsampNgainVariant=Passthrough  TsampIntegralVariant=Disabled_SignalSpec  ExternalSaturationOutDataTypeStr=Inherit: Same as second input  DerivativeSourceVariant=Disabled  PreIntVariant=InternalPreInt
  Sum : Sum  Inputs=|+-
  M_w : Outport
  wires:
  Constant/1 -> Sum/2
  Sum/1 -> PID Controller/1  "err"
  tank/1 -> Sum/1
  PID Controller/1 -> M_w/1

== system microturbine_model_v2/Heat Recovery Boiler/Tank ==
  m w : Inport
  T8 : Inport  Port=2
  Gain : Gain  Gain=1/M_buffer
  Integrator : Integrator  InitialCondition=hot_water_setpoint
  Product : Product
  Subtract : Sum  Inputs=-+
  T_tank : Outport
  wires:
  Gain/1 -> Product/2
  Product/1 -> Integrator/1
  Integrator/1 -> T_tank/1, Subtract/1  "T_tank"
  Subtract/1 -> Product/1
  m w/1 -> Gain/1
  T8/1 -> Subtract/2

== matlab function microturbine_model_v2/Compressor/MATLAB Function ==
  settings: updateMethod=DISCRETE  sampleTime=0.4
  data: beta input; m input
function updatePlot(beta, m)
    coder.extrinsic('updateCompressorMap');   % run as plain MATLAB, not generated code
    updateCompressorMap(m, beta);
end

== matlab function microturbine_model_v2/Turbine/MATLAB Function ==
  data: P3 input; P4 input; T3 input; T4_prime output; eta_t input; k input; t input
function T4_prime = turbine(P3, P4, T3, eta_t, k, t)
    beta = P3 / P4;
    beta_crit = ((k+1)/2)^(k/(k-1));

    if beta < beta_crit || ~isfinite(beta)
        warning('MT:turbineNotChoked', 't=%.4f: Turbine not choked: beta=%.3f (crit=%.3f). Choking assumption invalid.', t, beta, beta_crit);
        beta = beta_crit;   % clamp during invalid transients, avoids complex power()
    end
    
    n = (k-1)/k;
    T4_prime = T3 - eta_t * T3 * ( 1 - 1 / ( beta^n ) );
end

== matlab function microturbine_model_v2/Load limiter/Upper limit ==
  data: Pprod input; Up output; Pmax input
function Up = rateLim(Pprod, Pmax)

    if Pprod <= 0.5*Pmax
        Up = 1000;
    elseif Pprod <= 0.7*Pmax
        Up = 700;
    elseif Pprod <= 0.75*Pmax
        Up = 500;
    elseif Pprod <= 0.8*Pmax
        Up = 250;
    elseif Pprod <= 0.85*Pmax
        Up = 200;
    else
        Up = 150;        
    end
end

== matlab function microturbine_model_v2/Fuel control/MATLAB Function ==
  data: m_f_max_dyn output; M_x input; T3_max input; T3_min input; T2pp input; c_p_air input; c_p_eg input; LHV input; eta_comb input; m_f_min_dyn output
function [m_f_max_dyn, m_f_min_dyn] = maxFuel(M_x, T3_max, T3_min, T2pp, ...
    c_p_air, c_p_eg, LHV, eta_comb)

m_f_max_dyn = max(0, M_x*(c_p_eg*T3_max - c_p_air*T2pp) ...
    /(LHV*eta_comb - c_p_eg*T3_max));

m_f_min_dyn = max(0, M_x*(c_p_eg*T3_min - c_p_air*T2pp) ...
    /(LHV*eta_comb - c_p_eg*T3_min));

end

== matlab function microturbine_model_v2/Recuperator/MATLAB Function1 ==
  data: Qc output; Tm input; T2pp output; m_a input; T2p input; UAc0 input; ma0 input; cpa input
function [Qc, T2pp] = recCold(Tm, m_a, T2p, UAc0, ma0, cpa)
N   = 5;
Cc  = max(m_a*cpa, 1);
UAc = UAc0 * (max(m_a,1e-3)/ma0)^0.8;
ec  = exp(-(UAc/N)/Cc);
Qc  = zeros(N,1);
t   = T2p;
for i = 1:N
    o = Tm(i) + (t - Tm(i))*ec;
    Qc(i) = Cc*(o - t);
    t = o;
end
T2pp = t;
end

== matlab function microturbine_model_v2/Compressor/MATLAB Function1 ==
  data: T1 input; P1 input; P2 input; T2_prime output; k input; eta_c input
function T2_prime = adiabaticCompression(T1, P1, P2, k, eta_c)
    
    beta = P2 / P1;

    if beta < 0
        error('Negative beta. beta=%.2f, P1=%.0f, P2=%.0f', beta, P1, P2);
    end

    T2_prime = T1 * ( 1 + ( (beta)^( (k-1) / k ) - 1 ) / eta_c );

end

== matlab function microturbine_model_v2/Recuperator/MATLAB Function2 ==
  data: Tm input; T5 output; m_eg input; T4p input; UAh0 input; meg0 input; cpe input; Qh output
function [T5, Qh] = recHot(Tm, m_eg, T4p, UAh0, meg0, cpe)
N   = 5;
Ch  = max(m_eg*cpe, 1);
UAh = UAh0 * (max(m_eg,1e-3)/meg0)^0.8;
eh  = exp(-(UAh/N)/Ch);
Qh  = zeros(N,1);
t   = T4p;
for i = N:-1:1
    o = Tm(i) + (t - Tm(i))*eh;
    Qh(i) = Ch*(t - o);
    t = o;
end
T5 = t;
end
